simulink model "ISTrain_2024"  (R2024b)
settings: Solver=ode4  StartTime=0.0  StopTime=StopTime  FixedStep=StepSize  RelTol=1e-3
undefined symbols (not defined in the file or in its folder): Crr, eta_mech, g, G, grade, LM, LMatrix, LR, m_loco, m_total, maxID, maxIQ, maxTorque, Pp, r_w, RLInv, Rr
libraries: slpidlib x3
settings Model: Creator=rafae  LastModifiedBy=rafae

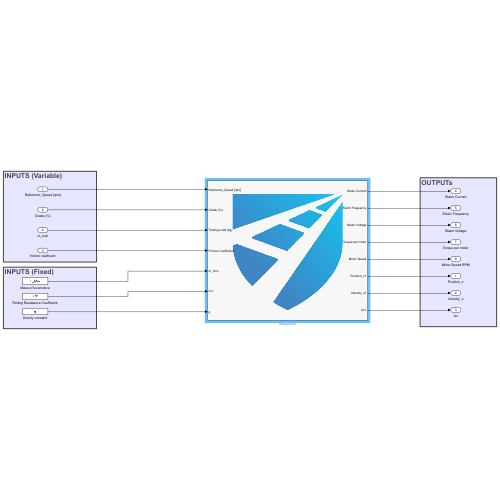
[thumbnail: Simulink's stored preview of the top-level diagram]
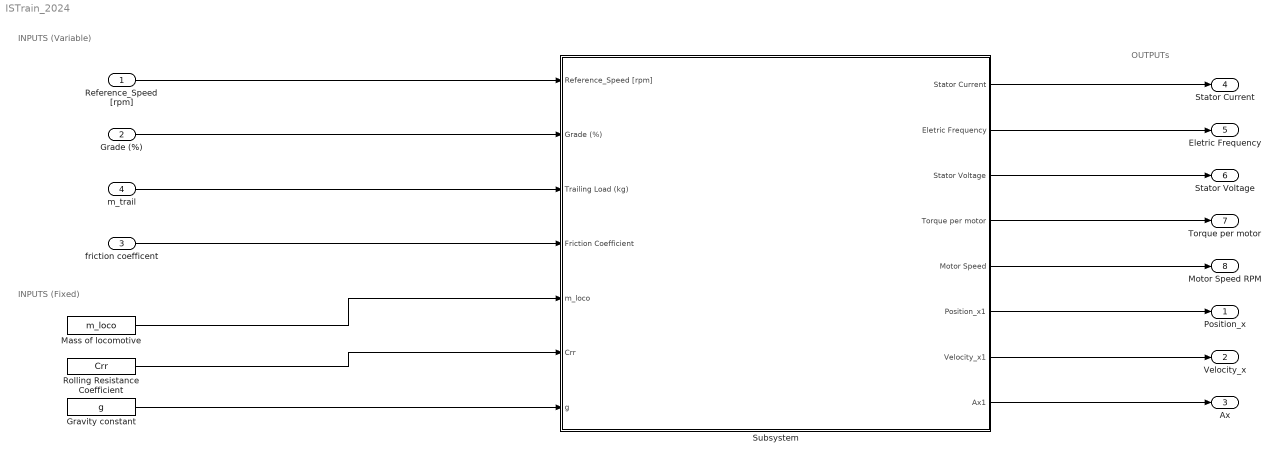
== system ISTrain_2024 ==
  note: OUTPUTs
  note: INPUTS (Variable)
  note: INPUTS (Fixed)
  Reference_Speed [rpm] : Inport
  Grade (%) : Inport  Port=2
  friction coefficent : Inport  Port=3
  m_trail : Inport  Port=4
  Gravity constant : Constant  Value=g
  Mass of locomotive : Constant  Value=m_loco
  Rolling Resistance Coefficient : Constant  Value=Crr
  Subsystem : Subsystem
      mask Display: image('ist_train_logo.jpg');
  Position_x : Outport
  Velocity_x : Outport  Port=2
  Ax : Outport  Port=3
  Stator Current : Outport  Port=4
  Eletric Frequency : Outport  Port=5
  Stator Voltage : Outport  Port=6
  Torque per motor : Outport  Port=7
  Motor Speed RPM : Outport  Port=8
  wires:
  Reference_Speed [rpm]/1 -> Subsystem/1(Reference_Speed [rpm])
  Subsystem/6(Position_x1) -> Position_x/1
  Subsystem/7(Velocity_x1) -> Velocity_x/1
  Subsystem/8(Ax1) -> Ax/1
  Subsystem/1(Stator Current) -> Stator Current/1
  Subsystem/2(Eletric Frequency) -> Eletric Frequency/1
  Subsystem/3(Stator Voltage) -> Stator Voltage/1
  Subsystem/4(Torque per motor) -> Torque per motor/1
  Subsystem/5(Motor Speed) -> Motor Speed RPM/1
  Grade (%)/1 -> Subsystem/2(Grade (%))
  m_trail/1 -> Subsystem/3(Trailing Load (kg))
  friction coefficent/1 -> Subsystem/4(Friction Coefficient)
  Mass of locomotive/1 -> Subsystem/5(m_loco)
  Rolling Resistance Coefficient/1 -> Subsystem/6(Crr)
  Gravity constant/1 -> Subsystem/7(g)

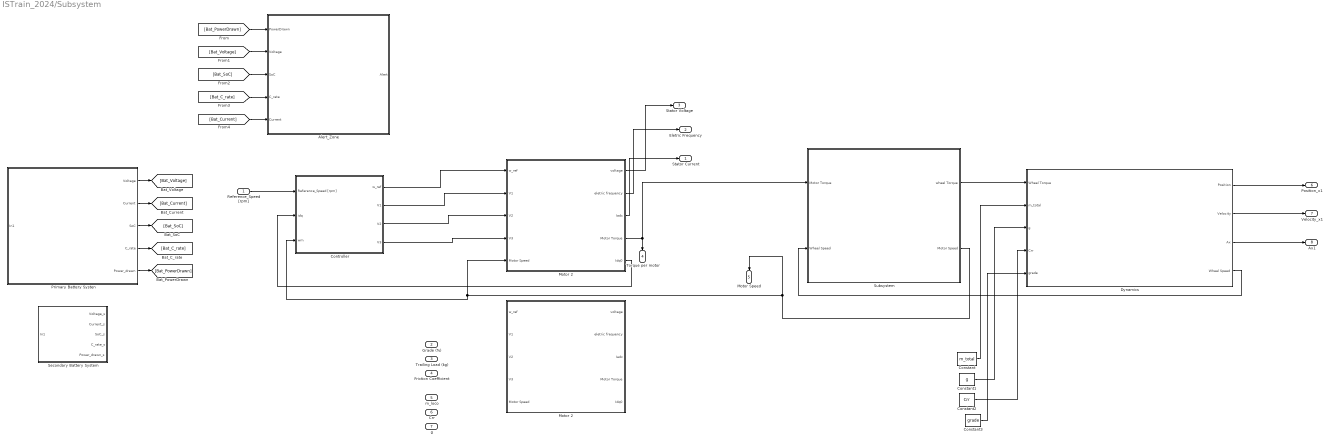
== system ISTrain_2024/Subsystem ==
  Reference_Speed [rpm] : Inport
  Grade (%) : Inport  Port=2
  Trailing Load (kg) : Inport  Port=3
  Friction Coefficient : Inport  Port=4
  m_loco : Inport  Port=5
  Crr : Inport  Port=6
  g : Inport  Port=7
  Alert_Zone : Subsystem
      mask Display: image('hazard.jpg');
  Constant : Constant  Value=m_total
  Constant1 : Constant  Value=g
  Constant2 : Constant  Value=Crr
  Constant3 : Constant  Value=grade
  Controller : Subsystem
      mask Display: image('motor controller.jpeg');
  Dynamics : Subsystem
      mask Display: image('wheel_train.jpg');
  Motor 2 : Subsystem
      mask Display: image('motor.jpg');
  "Motor 2 " : Subsystem
      mask Display: image('motor.jpg');
  Primary Battery Systen : Subsystem
      mask Display: image('battery system.png');
  Secondary Battery System : Subsystem
      mask Display: image('battery system.png');
  Subsystem : Subsystem
      mask Display: image('gear_system.png');
  Stator Current : Outport
  Eletric Frequency : Outport  Port=2
  Stator Voltage : Outport  Port=3
  Torque per motor : Outport  Port=4
  Motor Speed : Outport  Port=5
  Position_x1 : Outport  Port=6
  Velocity_x1 : Outport  Port=7
  Ax1 : Outport  Port=8
  wires:
  Reference_Speed [rpm]/1 -> Controller/1(Reference_Speed [rpm])
  Subsystem/2(Motor Speed) -> Motor Speed/1, Controller/3(wm), "Motor 2 "/5(Motor Speed)
  Dynamics/4(Wheel Speed) -> Subsystem/2(Wheel Speed)
  Controller/1(w_ref) -> "Motor 2 "/1(w_ref)
  Controller/2(V1) -> "Motor 2 "/2(V1)
  Controller/3(V2) -> "Motor 2 "/3(V2)
  Controller/4(V3) -> "Motor 2 "/4(V3)
  "Motor 2 "/5(Idq0) -> Controller/2(idq)
  "Motor 2 "/1(voltage) -> Stator Voltage/1
  "Motor 2 "/2(eletric frequency) -> Eletric Frequency/1
  "Motor 2 "/3(Iadc) -> Stator Current/1
  "Motor 2 "/4(Motor Torque) -> Subsystem/1(Motor Torque), Torque per motor/1
  Subsystem/1(wheel Torque) -> Dynamics/1(Wheel Torque)
  Constant3/1 -> Dynamics/5(grade)
  Constant1/1 -> Dynamics/3(g)
  Constant2/1 -> Dynamics/4(Crr)
  Constant/1 -> Dynamics/2(m_total)
  Dynamics/3(Ax) -> Ax1/1
  Dynamics/2(Velocity) -> Velocity_x1/1
  Dynamics/1(Position) -> Position_x1/1
  Primary Battery Systen/1(Voltage) -> [Bat_Voltage]
  Primary Battery Systen/2(Current) -> [Bat_Current]
  Primary Battery Systen/3(SoC) -> [Bat_SoC]
  Primary Battery Systen/5(Power_drawn) -> [Bat_PowerDrawn]
  Primary Battery Systen/4(C_rate) -> [Bat_C_rate]
  [Bat_Current] -> Alert_Zone/5(Current)
  [Bat_C_rate] -> Alert_Zone/4(C_rate)
  [Bat_SoC] -> Alert_Zone/3(SoC)
  [Bat_Voltage] -> Alert_Zone/2(Voltage)
  [Bat_PowerDrawn] -> Alert_Zone/1(PowerDrawn)

== system ISTrain_2024/Subsystem/Alert_Zone ==
  PowerDrawn : Inport
  Voltage : Inport  Port=2
  SoC : Inport  Port=3
  C_rate : Inport  Port=4
  Current : Inport  Port=5
  MATLAB Function : MATLAB Function  TreatAsAtomicUnit=on
  Alert : Outport
  wires:
  Voltage/1 -> MATLAB Function/2(Voltage)
  SoC/1 -> MATLAB Function/1(SoC)
  MATLAB Function/1(alert) -> Alert/1
  C_rate/1 -> MATLAB Function/3(C_rate)

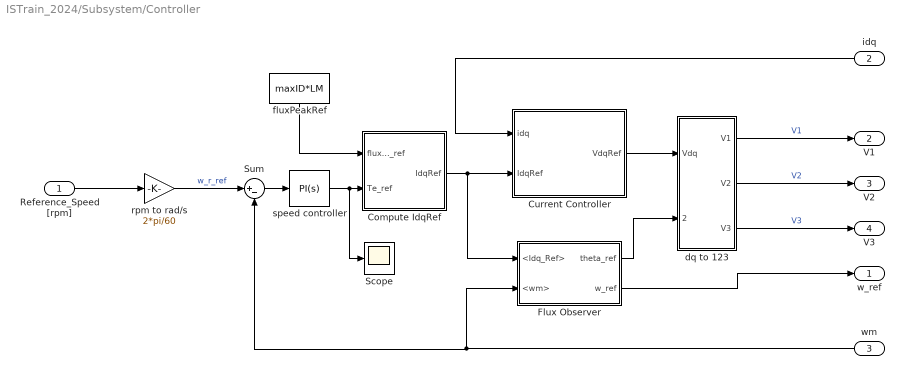
== system ISTrain_2024/Subsystem/Controller ==
  Reference_Speed [rpm] : Inport
  idq : Inport  Port=2
  wm : Inport  Port=3
  Compute IdqRef : Subsystem
  Current Controller : Subsystem
  Flux Observer : Subsystem
  Scope : Scope
  Sum : Sum  Inputs=|+-
  dq to 123 : Subsystem
  fluxPeakRef : Constant  Value=maxID*LM
  rpm to rad/s : Gain  Gain=2*pi/60
  speed controller : slpidlib/PID Controller  Controller=PI  Form=Parallel  TimeDomain=Continuous-time  UseExternalTs=off  SampleTime=-1  IntegratorMethod=Forward Euler  FilterMethod=Forward Euler  ControllerParametersSource=internal  P=50  I=100  UseKiTs=off  D=0  UseExternalDerivativeSource=off  N=100  UseFilter=on  TunerSelectOption=Transfer Function Based (PID Tuner App)  InitialConditionSource=internal  InitialConditionForIntegrator=0  InitialConditionForFilter=0  DifferentiatorICPrevScaledInput=0  ExternalReset=none  TrackingMode=off  Kt=1  LimitOutput=on  SatLimitsSource=internal  UpperSaturationLimit=maxTorque  LowerSaturationLimit=-maxTorque  LinearizeAsGain=on  AntiWindupMode=back-calculation  Kb=500  LimitIntegrator=off  UpperIntegratorSaturationLimit=inf  LowerIntegratorSaturationLimit=-inf  POutMin=[]  POutMax=[]  IOutMin=[]  IOutMax=[]  DOutMin=[]  DOutMax=[]  NOutMin=[]  NOutMax=[]  SumOutMin=[]  SumOutMax=[]  SaturationOutMin=[]  SaturationOutMax=[]  PParamMin=[]  PParamMax=[]  IParamMin=[]  IParamMax=[]  DParamMin=[]  DParamMax=[]  NParamMin=[]  NParamMax=[]  KbParamMin=[]  KbParamMax=[]  KtParamMin=[]  KtParamMax=[]  KbOutMin=[]  KbOutMax=[]  KtOutMin=[]  KtOutMax=[]  IntegratorOutMin=[]  IntegratorOutMax=[]  FilterOutMin=[]  FilterOutMax=[]  SumI1OutMin=[]  SumI1OutMax=[]  SumI2OutMin=[]  SumI2OutMax=[]  SumI3OutMin=[]  SumI3OutMax=[]  SumI4OutMin=[]  SumI4OutMax=[]  SumDOutMin=[]  SumDOutMax=[]  DifferentiatorOutMin=[]  DifferentiatorOutMax=[]  FilterDiffOutCoefMin=[]  FilterDiffOutCoefMax=[]  ReciprocalOutMin=[]  ReciprocalOutMax=[]  SumDenOutMin=[]  SumDenOutMax=[]  SumNumOutMin=[]  SumNumOutMax=[]  DivideOutMin=[]  DivideOutMax=[]  UdiffTsProdOutMin=[]  UdiffTsProdOutMax=[]  NTsProdOutMin=[]  NTsProdOutMax=[]  UintegralTsProdOutMin=[]  UintegralTsProdOutMax=[]  UngainTsProdOutMin=[]  UngainTsProdOutMax=[]  ClampingZeroOutDataTypeStr=Inherit: Inherit via back propagation  ClampingZeroOutMin=[]  ClampingZeroOutMax=[]  FilterDenConstantOutDataTypeStr=Inherit: Inherit via back propagation  FilterDenConstantOutMin=[]  FilterDenConstantOutMax=[]  PCopyOutDataTypeStr=Inherit: Inherit via back propagation  PCopyOutMin=[]  PCopyOutMax=[]  NCopyOutDataTypeStr=Inherit: Inherit via back propagation  NCopyOutMin=[]  NCopyOutMax=[]  IntegratorContinuousStateAttributes=''  IntegratorStateMustResolveToSignalObject=off  IntegratorRTWStateStorageClass=Auto  FilterContinuousStateAttributes=''  FilterStateMustResolveToSignalObject=off  FilterRTWStateStorageClass=Auto  ParallelPVariant=InternalParameters  IdealPVariant=Disabled  IVariant=InternalParameters  DVariant=Disabled  IntegratorVariant=Continuous  SatVariant=Enabled  AWVariant=BackCalculation  PCopyVariant=Disabled  TRVariant=Disabled  FdbkBlocksVariant=Forward  IdealPFdbkVariant=Disabled  SatFdbkVariant=Disabled  DerivativeFilterVariant=Disabled  NVariant=Disabled  NCopyVariant=Disabled_SignalSpec  FilterICVariant=Disabled  IntegratorICVariant=InternalICs  ExternalResetVariant=Disabled  TRSumVariant=Passthrough  SumFdbkVariant=Disabled  SumVariant=Sum_PI  TsampFilterVariant=InternalTs  TsampNgainVariant=Passthrough  TsampIntegralVariant=Disabled_SignalSpec  ExternalSaturationOutDataTypeStr=Inherit: Same as second input  DerivativeSourceVariant=Disabled  PreIntVariant=InternalPreInt
  w_ref : Outport  VectorParamsAs1DForOutWhenUnconnected=off
  V1 : Outport  Port=2  VectorParamsAs1DForOutWhenUnconnected=off
  V2 : Outport  Port=3  VectorParamsAs1DForOutWhenUnconnected=off
  V3 : Outport  Port=4  VectorParamsAs1DForOutWhenUnconnected=off
  wires:
  Compute IdqRef/1(IdqRef) -> Flux Observer/1(<Idq_Ref>), Current Controller/2(IdqRef)
  Sum/1 -> speed controller/1
  fluxPeakRef/1 -> Compute IdqRef/1(fluxdR_ref)
  dq to 123/3(V3) -> V3/1  "V3"
  wm/1 -> Sum/2, Flux Observer/2(<wm>)
  speed controller/1 -> Scope/1, Compute IdqRef/2(Te_ref)
  idq/1 -> Current Controller/1(idq)
  Reference_Speed [rpm]/1 -> rpm to rad/s/1
  dq to 123/2(V2) -> V2/1  "V2"
  dq to 123/1(V1) -> V1/1  "V1"
  rpm to rad/s/1 -> Sum/1  "w_r_ref"
  Flux Observer/2(w_ref) -> w_ref/1
  Flux Observer/1(theta_ref) -> dq to 123/2(theta_ref)
  Current Controller/1(VdqRef) -> dq to 123/1(Vdq)

== system ISTrain_2024/Subsystem/Dynamics ==
  Wheel Torque : Inport
  m_total : Inport  Port=2
  g : Inport  Port=3
  Crr : Inport  Port=4
  grade : Inport  Port=5
  Gain : Gain  Gain=1/(m_total)
  Gain1 : Gain  Gain=1/r_w
  Integrator : Integrator
  Integrator1 : Integrator
  MATLAB Function : MATLAB Function  TreatAsAtomicUnit=on
  Subtract : Sum  Inputs=+-
  Position : Outport
  Velocity : Outport  Port=2
  Ax : Outport  Port=3
  Wheel Speed : Outport  Port=4
  wires:
  Integrator1/1 -> Position/1
  grade/1 -> MATLAB Function/4(grade)
  Crr/1 -> MATLAB Function/3(Crr)
  Subtract/1 -> Gain/1
  Integrator/1 -> Gain1/1, Velocity/1, Integrator1/1
  MATLAB Function/1(F_res) -> Subtract/2
  m_total/1 -> MATLAB Function/1(m_total)
  g/1 -> MATLAB Function/2(g)
  Gain1/1 -> Wheel Speed/1
  Gain/1 -> Ax/1, Integrator/1
  Wheel Torque/1 -> Subtract/1

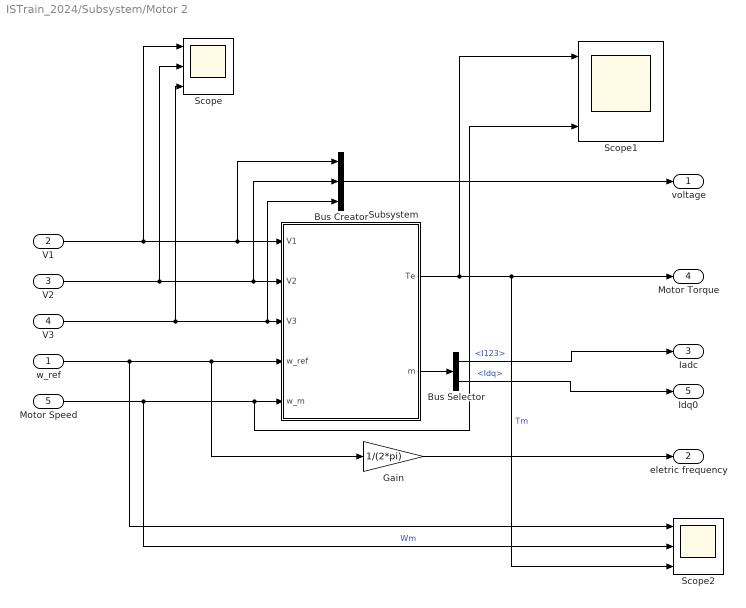
== system ISTrain_2024/Subsystem/Motor 2 ==
  w_ref : Inport
  V1 : Inport  Port=2
  V2 : Inport  Port=3
  V3 : Inport  Port=4
  Motor Speed : Inport  Port=5
  Bus Creator : BusCreator  Inputs=3
  Bus Selector : BusSelector  OutputSignals=I123,Idq
  Gain : Gain  Gain=1/(2*pi)
  Scope : Scope  NumInputPorts=3
  Scope1 : Scope  NumInputPorts=3
  Scope2 : Scope  NumInputPorts=3
  Subsystem : Subsystem
  voltage : Outport  VectorParamsAs1DForOutWhenUnconnected=off
  eletric frequency : Outport  Port=2  VectorParamsAs1DForOutWhenUnconnected=off
  Iadc : Outport  Port=3  VectorParamsAs1DForOutWhenUnconnected=off
  Motor Torque : Outport  Port=4  VectorParamsAs1DForOutWhenUnconnected=off
  Idq0 : Outport  Port=5  VectorParamsAs1DForOutWhenUnconnected=off
  wires:
  Gain/1 -> eletric frequency/1
  Subsystem/1(Te) -> Scope1/1, Scope2/3, Motor Torque/1  "Tm"
  Bus Selector/2 -> Idq0/1  "<Idq>"
  Subsystem/2(m) -> Bus Selector/1
  Bus Creator/1 -> voltage/1
  V1/1 -> Bus Creator/1, Subsystem/1(V1), Scope/1
  Motor Speed/1 -> Scope2/2, Scope1/3, Subsystem/5(w_m)  "Wm"
  Bus Selector/1 -> Iadc/1  "<I123>"
  w_ref/1 -> Scope2/1, Gain/1, Subsystem/4(w_ref)
  V2/1 -> Bus Creator/2, Subsystem/2(V2), Scope/2
  V3/1 -> Scope/3, Bus Creator/3, Subsystem/3(V3)

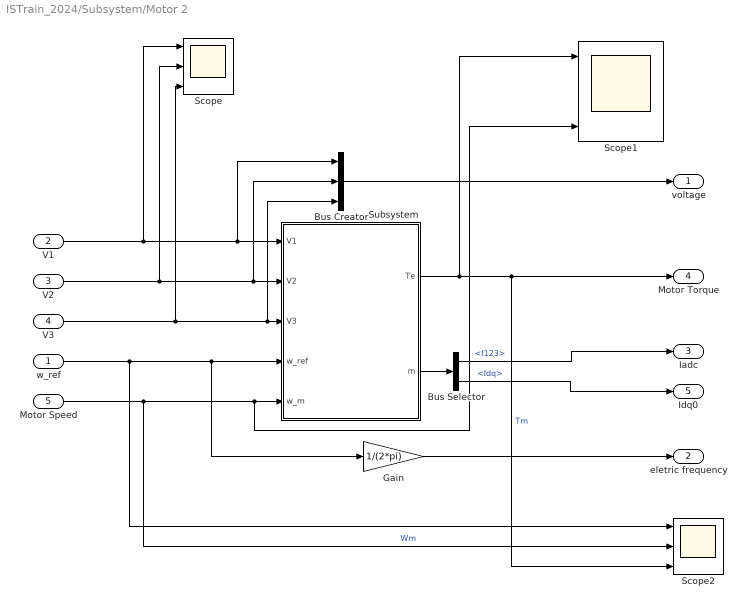
== system ISTrain_2024/Subsystem/Motor 2  ==
  w_ref : Inport
  V1 : Inport  Port=2
  V2 : Inport  Port=3
  V3 : Inport  Port=4
  Motor Speed : Inport  Port=5
  Bus Creator : BusCreator  Inputs=3
  Bus Selector : BusSelector  OutputSignals=I123,Idq
  Gain : Gain  Gain=1/(2*pi)
  Scope : Scope  NumInputPorts=3
  Scope1 : Scope  NumInputPorts=3
  Scope2 : Scope  NumInputPorts=3
  Subsystem : Subsystem
  voltage : Outport  VectorParamsAs1DForOutWhenUnconnected=off
  eletric frequency : Outport  Port=2  VectorParamsAs1DForOutWhenUnconnected=off
  Iadc : Outport  Port=3  VectorParamsAs1DForOutWhenUnconnected=off
  Motor Torque : Outport  Port=4  VectorParamsAs1DForOutWhenUnconnected=off
  Idq0 : Outport  Port=5  VectorParamsAs1DForOutWhenUnconnected=off
  wires:
  Gain/1 -> eletric frequency/1
  Subsystem/1(Te) -> Scope1/1, Scope2/3, Motor Torque/1  "Tm"
  Bus Selector/2 -> Idq0/1  "<Idq>"
  Subsystem/2(m) -> Bus Selector/1
  Bus Creator/1 -> voltage/1
  V1/1 -> Bus Creator/1, Subsystem/1(V1), Scope/1
  Motor Speed/1 -> Scope2/2, Scope1/3, Subsystem/5(w_m)  "Wm"
  Bus Selector/1 -> Iadc/1  "<I123>"
  w_ref/1 -> Scope2/1, Gain/1, Subsystem/4(w_ref)
  V2/1 -> Bus Creator/2, Subsystem/2(V2), Scope/2
  V3/1 -> Scope/3, Bus Creator/3, Subsystem/3(V3)

== system ISTrain_2024/Subsystem/Primary Battery Systen ==
  In1 : Inport
  From Workspace : FromWorkspace  VariableName=power_signal
  MATLAB Function : MATLAB Function  TreatAsAtomicUnit=on
  Scope : Scope  NumInputPorts=5
  Voltage : Outport
  Current : Outport  Port=2
  SoC : Outport  Port=3
  C_rate : Outport  Port=4
  Power_drawn : Outport  Port=5
  wires:
  From Workspace/1 -> MATLAB Function/1(P_in)
  MATLAB Function/1(V_out) -> Scope/1, Voltage/1
  MATLAB Function/2(I_out) -> Scope/2, Current/1
  MATLAB Function/3(SoC_out) -> Scope/3, SoC/1
  MATLAB Function/4(C_out) -> Scope/4, C_rate/1
  MATLAB Function/5(P_out) -> Scope/5, Power_drawn/1

== system ISTrain_2024/Subsystem/Secondary Battery System ==
  In1 : Inport
  Voltage_s : Outport
  Current_s : Outport  Port=2
  SoC_s : Outport  Port=3
  C_rate_s : Outport  Port=4
  Power_drawn_s : Outport  Port=5

== system ISTrain_2024/Subsystem/Subsystem ==
  Motor Torque : Inport
  Wheel Speed : Inport  Port=2
  GearBox : Subsystem
  wheel Torque : Outport
  Motor Speed : Outport  Port=2
  wires:
  Motor Torque/1 -> GearBox/1(Torque total)
  Wheel Speed/1 -> Motor Speed/1
  GearBox/1(Tractive_Force) -> wheel Torque/1

== system ISTrain_2024/Subsystem/Controller/Compute IdqRef ==
  fluxdR_ref : Inport
  Te_ref : Inport  Port=2
  Fcn : Fcn  Expr=u(2)/(3/2*Pp*(LM/LR)*u(1))
  Gain : Gain  Gain=1/LM
  Mux : Mux  Inputs=2
  Mux1 : Mux  Inputs=2
  Saturation : Saturate  UpperLimit=maxID  LowerLimit=-maxID
  Saturation1 : Saturate  UpperLimit=maxIQ  LowerLimit=-maxIQ
  IdqRef : Outport  VectorParamsAs1DForOutWhenUnconnected=off
  wires:
  fluxdR_ref/1 -> Mux/1, Gain/1
  Mux/1 -> Fcn/1
  Fcn/1 -> Saturation1/1
  Gain/1 -> Saturation/1
  Mux1/1 -> IdqRef/1
  Te_ref/1 -> Mux/2
  Saturation/1 -> Mux1/1  "id"
  Saturation1/1 -> Mux1/2  "iq"

== system ISTrain_2024/Subsystem/Controller/Current Controller ==
  idq : Inport
  IdqRef : Inport  Port=2
  Demux : Demux  Outputs=2
  Mux : Mux  Inputs=2
  PID Controller : slpidlib/PID Controller  Controller=PI  Form=Parallel  TimeDomain=Continuous-time  UseExternalTs=off  SampleTime=-1  IntegratorMethod=Forward Euler  FilterMethod=Forward Euler  ControllerParametersSource=internal  P=5  I=100  UseKiTs=off  D=0  UseExternalDerivativeSource=off  N=100  UseFilter=on  TunerSelectOption=Transfer Function Based (PID Tuner App)  InitialConditionSource=internal  InitialConditionForIntegrator=0  InitialConditionForFilter=0  DifferentiatorICPrevScaledInput=0  ExternalReset=none  TrackingMode=off  Kt=1  LimitOutput=on  SatLimitsSource=internal  UpperSaturationLimit=600  LowerSaturationLimit=-600  LinearizeAsGain=on  AntiWindupMode=back-calculation  Kb=1  LimitIntegrator=off  UpperIntegratorSaturationLimit=inf  LowerIntegratorSaturationLimit=-inf  POutMin=[]  POutMax=[]  IOutMin=[]  IOutMax=[]  DOutMin=[]  DOutMax=[]  NOutMin=[]  NOutMax=[]  SumOutMin=[]  SumOutMax=[]  SaturationOutMin=[]  SaturationOutMax=[]  PParamMin=[]  PParamMax=[]  IParamMin=[]  IParamMax=[]  DParamMin=[]  DParamMax=[]  NParamMin=[]  NParamMax=[]  KbParamMin=[]  KbParamMax=[]  KtParamMin=[]  KtParamMax=[]  KbOutMin=[]  KbOutMax=[]  KtOutMin=[]  KtOutMax=[]  IntegratorOutMin=[]  IntegratorOutMax=[]  FilterOutMin=[]  FilterOutMax=[]  SumI1OutMin=[]  SumI1OutMax=[]  SumI2OutMin=[]  SumI2OutMax=[]  SumI3OutMin=[]  SumI3OutMax=[]  SumI4OutMin=[]  SumI4OutMax=[]  SumDOutMin=[]  SumDOutMax=[]  DifferentiatorOutMin=[]  DifferentiatorOutMax=[]  FilterDiffOutCoefMin=[]  FilterDiffOutCoefMax=[]  ReciprocalOutMin=[]  ReciprocalOutMax=[]  SumDenOutMin=[]  SumDenOutMax=[]  SumNumOutMin=[]  SumNumOutMax=[]  DivideOutMin=[]  DivideOutMax=[]  UdiffTsProdOutMin=[]  UdiffTsProdOutMax=[]  NTsProdOutMin=[]  NTsProdOutMax=[]  UintegralTsProdOutMin=[]  UintegralTsProdOutMax=[]  UngainTsProdOutMin=[]  UngainTsProdOutMax=[]  ClampingZeroOutDataTypeStr=Inherit: Inherit via back propagation  ClampingZeroOutMin=[]  ClampingZeroOutMax=[]  FilterDenConstantOutDataTypeStr=Inherit: Inherit via back propagation  FilterDenConstantOutMin=[]  FilterDenConstantOutMax=[]  PCopyOutDataTypeStr=Inherit: Inherit via back propagation  PCopyOutMin=[]  PCopyOutMax=[]  NCopyOutDataTypeStr=Inherit: Inherit via back propagation  NCopyOutMin=[]  NCopyOutMax=[]  IntegratorContinuousStateAttributes=''  IntegratorStateMustResolveToSignalObject=off  IntegratorRTWStateStorageClass=Auto  FilterContinuousStateAttributes=''  FilterStateMustResolveToSignalObject=off  FilterRTWStateStorageClass=Auto  ParallelPVariant=InternalParameters  IdealPVariant=Disabled  IVariant=InternalParameters  DVariant=Disabled  IntegratorVariant=Continuous  SatVariant=Enabled  AWVariant=BackCalculation  PCopyVariant=Disabled  TRVariant=Disabled  FdbkBlocksVariant=Forward  IdealPFdbkVariant=Disabled  SatFdbkVariant=Disabled  DerivativeFilterVariant=Disabled  NVariant=Disabled  NCopyVariant=Disabled_SignalSpec  FilterICVariant=Disabled  IntegratorICVariant=InternalICs  ExternalResetVariant=Disabled  TRSumVariant=Passthrough  SumFdbkVariant=Disabled  SumVariant=Sum_PI  TsampFilterVariant=InternalTs  TsampNgainVariant=Passthrough  TsampIntegralVariant=Disabled_SignalSpec  ExternalSaturationOutDataTypeStr=Inherit: Same as second input  DerivativeSourceVariant=Disabled  PreIntVariant=InternalPreInt
  PID Controller1 : slpidlib/PID Controller  Controller=PI  Form=Parallel  TimeDomain=Continuous-time  UseExternalTs=off  SampleTime=-1  IntegratorMethod=Forward Euler  FilterMethod=Forward Euler  ControllerParametersSource=internal  P=5  I=100  UseKiTs=off  D=0  UseExternalDerivativeSource=off  N=100  UseFilter=on  TunerSelectOption=Transfer Function Based (PID Tuner App)  InitialConditionSource=internal  InitialConditionForIntegrator=0  InitialConditionForFilter=0  DifferentiatorICPrevScaledInput=0  ExternalReset=none  TrackingMode=off  Kt=1  LimitOutput=on  SatLimitsSource=internal  UpperSaturationLimit=600  LowerSaturationLimit=-600  LinearizeAsGain=on  AntiWindupMode=back-calculation  Kb=1  LimitIntegrator=off  UpperIntegratorSaturationLimit=inf  LowerIntegratorSaturationLimit=-inf  POutMin=[]  POutMax=[]  IOutMin=[]  IOutMax=[]  DOutMin=[]  DOutMax=[]  NOutMin=[]  NOutMax=[]  SumOutMin=[]  SumOutMax=[]  SaturationOutMin=[]  SaturationOutMax=[]  PParamMin=[]  PParamMax=[]  IParamMin=[]  IParamMax=[]  DParamMin=[]  DParamMax=[]  NParamMin=[]  NParamMax=[]  KbParamMin=[]  KbParamMax=[]  KtParamMin=[]  KtParamMax=[]  KbOutMin=[]  KbOutMax=[]  KtOutMin=[]  KtOutMax=[]  IntegratorOutMin=[]  IntegratorOutMax=[]  FilterOutMin=[]  FilterOutMax=[]  SumI1OutMin=[]  SumI1OutMax=[]  SumI2OutMin=[]  SumI2OutMax=[]  SumI3OutMin=[]  SumI3OutMax=[]  SumI4OutMin=[]  SumI4OutMax=[]  SumDOutMin=[]  SumDOutMax=[]  DifferentiatorOutMin=[]  DifferentiatorOutMax=[]  FilterDiffOutCoefMin=[]  FilterDiffOutCoefMax=[]  ReciprocalOutMin=[]  ReciprocalOutMax=[]  SumDenOutMin=[]  SumDenOutMax=[]  SumNumOutMin=[]  SumNumOutMax=[]  DivideOutMin=[]  DivideOutMax=[]  UdiffTsProdOutMin=[]  UdiffTsProdOutMax=[]  NTsProdOutMin=[]  NTsProdOutMax=[]  UintegralTsProdOutMin=[]  UintegralTsProdOutMax=[]  UngainTsProdOutMin=[]  UngainTsProdOutMax=[]  ClampingZeroOutDataTypeStr=Inherit: Inherit via back propagation  ClampingZeroOutMin=[]  ClampingZeroOutMax=[]  FilterDenConstantOutDataTypeStr=Inherit: Inherit via back propagation  FilterDenConstantOutMin=[]  FilterDenConstantOutMax=[]  PCopyOutDataTypeStr=Inherit: Inherit via back propagation  PCopyOutMin=[]  PCopyOutMax=[]  NCopyOutDataTypeStr=Inherit: Inherit via back propagation  NCopyOutMin=[]  NCopyOutMax=[]  IntegratorContinuousStateAttributes=''  IntegratorStateMustResolveToSignalObject=off  IntegratorRTWStateStorageClass=Auto  FilterContinuousStateAttributes=''  FilterStateMustResolveToSignalObject=off  FilterRTWStateStorageClass=Auto  ParallelPVariant=InternalParameters  IdealPVariant=Disabled  IVariant=InternalParameters  DVariant=Disabled  IntegratorVariant=Continuous  SatVariant=Enabled  AWVariant=BackCalculation  PCopyVariant=Disabled  TRVariant=Disabled  FdbkBlocksVariant=Forward  IdealPFdbkVariant=Disabled  SatFdbkVariant=Disabled  DerivativeFilterVariant=Disabled  NVariant=Disabled  NCopyVariant=Disabled_SignalSpec  FilterICVariant=Disabled  IntegratorICVariant=InternalICs  ExternalResetVariant=Disabled  TRSumVariant=Passthrough  SumFdbkVariant=Disabled  SumVariant=Sum_PI  TsampFilterVariant=InternalTs  TsampNgainVariant=Passthrough  TsampIntegralVariant=Disabled_SignalSpec  ExternalSaturationOutDataTypeStr=Inherit: Same as second input  DerivativeSourceVariant=Disabled  PreIntVariant=InternalPreInt
  Scope2 : Scope  NumInputPorts=2
  Sum1 : Sum  Inputs=+-
  VdqRef : Outport  VectorParamsAs1DForOutWhenUnconnected=off
  wires:
  IdqRef/1 -> Scope2/1, Sum1/1
  idq/1 -> Sum1/2
  PID Controller/1 -> Mux/1  "PI"
  Sum1/1 -> Scope2/2, Demux/1  "error"
  Demux/1 -> PID Controller/1
  Demux/2 -> PID Controller1/1
  PID Controller1/1 -> Mux/2
  Mux/1 -> VdqRef/1

== system ISTrain_2024/Subsystem/Controller/Flux Observer ==
  <Idq_Ref> : Inport
  <wm> : Inport  Port=2
  Add : Sum  Inputs=2
  Bias : Bias  Bias=+eps  SaturateOnIntegerOverflow=off
  Constant1 : Constant  Value=1/(LR/Rr)
  Demux : Demux  Outputs=2
  Gain : Gain  Gain=Pp
  Integrator : Integrator
  Product : Product  Inputs=*/
  Product1 : Product
  Selector : Selector  InputPortWidth=2  IndexOptions=Index vector (dialog)  Indices=[2 1]  OutputSizes=1
  theta_ref : Outport  VectorParamsAs1DForOutWhenUnconnected=off
  w_ref : Outport  Port=2  VectorParamsAs1DForOutWhenUnconnected=off
  wires:
  Demux/1 -> Product/1
  <wm>/1 -> Gain/1
  Constant1/1 -> Product1/1
  Selector/1 -> Demux/1
  Product1/1 -> Add/2
  Product/1 -> Product1/2
  <Idq_Ref>/1 -> Selector/1
  Add/1 -> w_ref/1, Integrator/1
  Bias/1 -> Product/2
  Demux/2 -> Bias/1
  Integrator/1 -> theta_ref/1
  Gain/1 -> Add/1

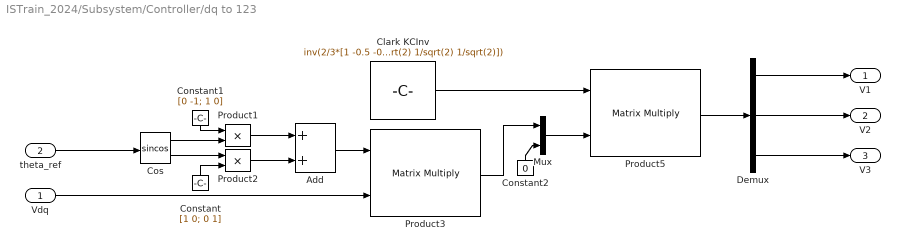
== system ISTrain_2024/Subsystem/Controller/dq to 123 ==
  Vdq : Inport
  theta_ref : Inport  Port=2
  Add : Sum
  Clark KCInv : Constant  Value=inv(2/3*[1 -0.5 -0.5; 0 sqrt(3)/2 -sqrt(3)/2; 1/sqrt(2) 1/sqrt(2) 1/sqrt(2)])
  Constant : Constant  Value=[1 0; 0 1]
  Constant1 : Constant  Value=[0 -1; 1 0]
  Constant2 : Constant  Value=0
  Cos : Trigonometry  Operator=sincos
  Demux : Demux  Outputs=3
  Mux : Mux  Inputs=2
  Product1 : Product
  Product2 : Product
  Product3 : Product  Multiplication=Matrix(*)
  Product5 : Product  Multiplication=Matrix(*)
  V1 : Outport  VectorParamsAs1DForOutWhenUnconnected=off
  V2 : Outport  Port=2  VectorParamsAs1DForOutWhenUnconnected=off
  V3 : Outport  Port=3  VectorParamsAs1DForOutWhenUnconnected=off
  wires:
  Cos/1 -> Product1/2
  Constant1/1 -> Product1/1
  Product2/1 -> Add/2
  Cos/2 -> Product2/1
  Product1/1 -> Add/1
  Constant/1 -> Product2/2
  Add/1 -> Product3/1
  Product3/1 -> Mux/1
  Clark KCInv/1 -> Product5/1
  Mux/1 -> Product5/2
  Constant2/1 -> Mux/2
  Vdq/1 -> Product3/2
  Demux/1 -> V1/1
  Demux/2 -> V2/1
  Demux/3 -> V3/1
  Product5/1 -> Demux/1
  theta_ref/1 -> Cos/1

== system ISTrain_2024/Subsystem/Motor 2/Subsystem ==
  note: V1 - phase-to-neutral voltage of phase 1 [V]
      | V2 - phase-to-neutral voltage of phase 2 [V]
      | V3 - phase-to-neutral voltage of phase 3 [V]
      | w_ref - reference of dq transformation (synchornous electric speed in this case = 2*pi*f) [rad/s]
      | w_m - motor angular speed [rad/s]
  V1 : Inport
  V2 : Inport  Port=2
  V3 : Inport  Port=3
  w_ref : Inport  Port=4
  w_m : Inport  Port=5
  Induction Machine Model : Subsystem
  Te : Outport  VectorParamsAs1DForOutWhenUnconnected=off
  m : Outport  Port=2  VectorParamsAs1DForOutWhenUnconnected=off
  wires:
  Induction Machine Model/1(m) -> m/1
  w_ref/1 -> Induction Machine Model/5(w_ref)
  V1/1 -> Induction Machine Model/2(V1)
  Induction Machine Model/2(Te) -> Te/1
  V2/1 -> Induction Machine Model/3(V2)
  V3/1 -> Induction Machine Model/4(V3)
  w_m/1 -> Induction Machine Model/1(wm)

== system ISTrain_2024/Subsystem/Motor 2 /Subsystem ==
  note: V1 - phase-to-neutral voltage of phase 1 [V]
      | V2 - phase-to-neutral voltage of phase 2 [V]
      | V3 - phase-to-neutral voltage of phase 3 [V]
      | w_ref - reference of dq transformation (synchornous electric speed in this case = 2*pi*f) [rad/s]
      | w_m - motor angular speed [rad/s]
  V1 : Inport
  V2 : Inport  Port=2
  V3 : Inport  Port=3
  w_ref : Inport  Port=4
  w_m : Inport  Port=5
  Induction Machine Model : Subsystem
  Te : Outport  VectorParamsAs1DForOutWhenUnconnected=off
  m : Outport  Port=2  VectorParamsAs1DForOutWhenUnconnected=off
  wires:
  Induction Machine Model/1(m) -> m/1
  w_ref/1 -> Induction Machine Model/5(w_ref)
  V1/1 -> Induction Machine Model/2(V1)
  Induction Machine Model/2(Te) -> Te/1
  V2/1 -> Induction Machine Model/3(V2)
  V3/1 -> Induction Machine Model/4(V3)
  w_m/1 -> Induction Machine Model/1(wm)

== system ISTrain_2024/Subsystem/Subsystem/GearBox ==
  Torque total : Inport
  Gear_ratio : Gain  Gain=G
  eta_mech : Gain  Gain=eta_mech
  Tractive_Force : Outport
  wires:
  Gear_ratio/1 -> eta_mech/1
  Torque total/1 -> Gear_ratio/1
  eta_mech/1 -> Tractive_Force/1

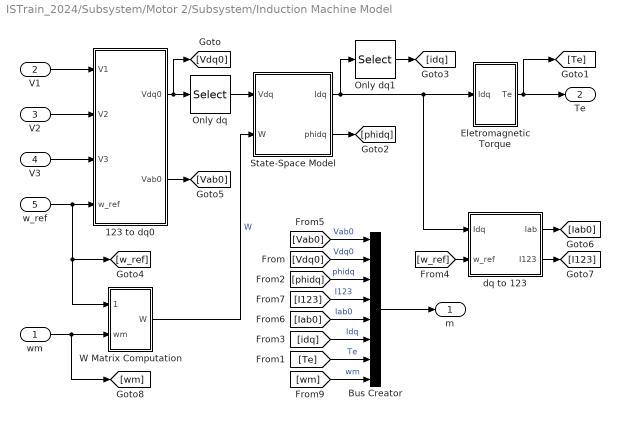
== system ISTrain_2024/Subsystem/Motor 2/Subsystem/Induction Machine Model ==
  wm : Inport
  V1 : Inport  Port=2
  V2 : Inport  Port=3
  V3 : Inport  Port=4
  w_ref : Inport  Port=5
  123 to dq0 : Subsystem
  Bus Creator : BusCreator  Inputs=8
  Eletromagnetic Torque : Subsystem
  Only dq : Selector  InputPortWidth=3  IndexOptions=Index vector (dialog)  Indices=[1 2]  OutputSizes=1
  Only dq1 : Selector  InputPortWidth=4  IndexOptions=Index vector (dialog)  Indices=[1 2]  OutputSizes=1
  State-Space Model : Subsystem
  W Matrix Computation : Subsystem
  dq to 123 : Subsystem
  m : Outport  VectorParamsAs1DForOutWhenUnconnected=off
  Te : Outport  Port=2  VectorParamsAs1DForOutWhenUnconnected=off
  wires:
  123 to dq0/1(Vdq0) -> Only dq/1, [Vdq0]
  V3/1 -> 123 to dq0/3(V3)
  V2/1 -> 123 to dq0/2(V2)
  wm/1 -> [wm], W Matrix Computation/2(wm)
  123 to dq0/2(Vab0) -> [Vab0]
  W Matrix Computation/1(W) -> State-Space Model/2(W)  "W"
  Only dq/1 -> State-Space Model/1(Vdq)
  Eletromagnetic Torque/1(Te) -> Te/1, [Te]
  V1/1 -> 123 to dq0/1(V1)
  State-Space Model/1(Idq) -> dq to 123/1(Idq), Eletromagnetic Torque/1(Idq), Only dq1/1
  [w_ref] -> dq to 123/2(w_ref)
  State-Space Model/2(phidq) -> [phidq]
  dq to 123/1(Iab) -> [Iab0]
  dq to 123/2(I123) -> [I123]
  [Vab0] -> Bus Creator/1  "Vab0"
  [Vdq0] -> Bus Creator/2  "Vdq0"
  [phidq] -> Bus Creator/3  "phidq"
  [I123] -> Bus Creator/4  "I123"
  [Iab0] -> Bus Creator/5  "Iab0"
  [idq] -> Bus Creator/6  "Idq"
  [Te] -> Bus Creator/7  "Te"
  Bus Creator/1 -> m/1
  Only dq1/1 -> [idq]
  w_ref/1 -> 123 to dq0/4(w_ref), W Matrix Computation/1(w_ref), [w_ref]
  [wm] -> Bus Creator/8  "wm"

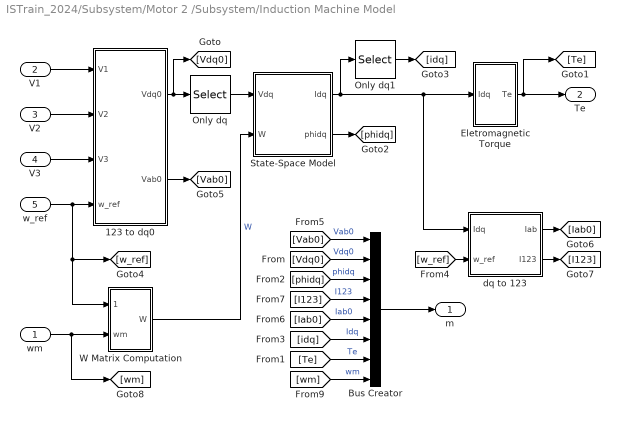
== system ISTrain_2024/Subsystem/Motor 2 /Subsystem/Induction Machine Model ==
  wm : Inport
  V1 : Inport  Port=2
  V2 : Inport  Port=3
  V3 : Inport  Port=4
  w_ref : Inport  Port=5
  123 to dq0 : Subsystem
  Bus Creator : BusCreator  Inputs=8
  Eletromagnetic Torque : Subsystem
  Only dq : Selector  InputPortWidth=3  IndexOptions=Index vector (dialog)  Indices=[1 2]  OutputSizes=1
  Only dq1 : Selector  InputPortWidth=4  IndexOptions=Index vector (dialog)  Indices=[1 2]  OutputSizes=1
  State-Space Model : Subsystem
  W Matrix Computation : Subsystem
  dq to 123 : Subsystem
  m : Outport  VectorParamsAs1DForOutWhenUnconnected=off
  Te : Outport  Port=2  VectorParamsAs1DForOutWhenUnconnected=off
  wires:
  123 to dq0/1(Vdq0) -> Only dq/1, [Vdq0]
  V3/1 -> 123 to dq0/3(V3)
  V2/1 -> 123 to dq0/2(V2)
  wm/1 -> [wm], W Matrix Computation/2(wm)
  123 to dq0/2(Vab0) -> [Vab0]
  W Matrix Computation/1(W) -> State-Space Model/2(W)  "W"
  Only dq/1 -> State-Space Model/1(Vdq)
  Eletromagnetic Torque/1(Te) -> Te/1, [Te]
  V1/1 -> 123 to dq0/1(V1)
  State-Space Model/1(Idq) -> dq to 123/1(Idq), Eletromagnetic Torque/1(Idq), Only dq1/1
  [w_ref] -> dq to 123/2(w_ref)
  State-Space Model/2(phidq) -> [phidq]
  dq to 123/1(Iab) -> [Iab0]
  dq to 123/2(I123) -> [I123]
  [Vab0] -> Bus Creator/1  "Vab0"
  [Vdq0] -> Bus Creator/2  "Vdq0"
  [phidq] -> Bus Creator/3  "phidq"
  [I123] -> Bus Creator/4  "I123"
  [Iab0] -> Bus Creator/5  "Iab0"
  [idq] -> Bus Creator/6  "Idq"
  [Te] -> Bus Creator/7  "Te"
  Bus Creator/1 -> m/1
  Only dq1/1 -> [idq]
  w_ref/1 -> 123 to dq0/4(w_ref), W Matrix Computation/1(w_ref), [w_ref]
  [wm] -> Bus Creator/8  "wm"

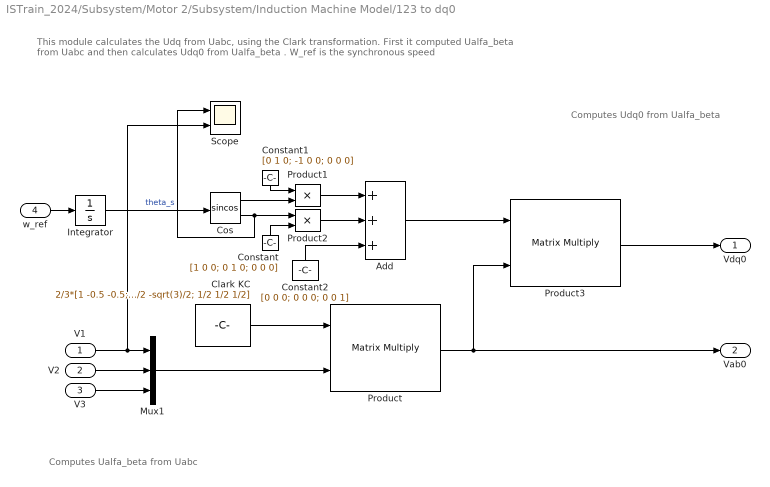
== system ISTrain_2024/Subsystem/Motor 2/Subsystem/Induction Machine Model/123 to dq0 ==
  note: Computes Ualfa_beta from Uabc
  note: This module calculates the Udq from Uabc, using the Clark transformation.
      | First it computed Ualfa_beta from Uabc and then calculates Udq0 from Ualfa_beta .
      | W_ref is the synchronous speed
  note: Computes Udq0 from Ualfa_beta
  V1 : Inport
  V2 : Inport  Port=2
  V3 : Inport  Port=3
  w_ref : Inport  Port=4
  Add : Sum  Inputs=+++
  Clark KC : Constant  Value=2/3*[1 -0.5 -0.5; 0 sqrt(3)/2 -sqrt(3)/2; 1/2 1/2 1/2]
  Constant : Constant  Value=[1 0 0; 0 1 0; 0 0 0]
  Constant1 : Constant  Value=[0 1 0; -1 0 0; 0 0 0]
  Constant2 : Constant  Value=[0 0 0; 0 0 0; 0 0 1]
  Cos : Trigonometry  Operator=sincos
  Integrator : Integrator
  Mux1 : Mux  Inputs=3
  Product : Product  Multiplication=Matrix(*)
  Product1 : Product
  Product2 : Product
  Product3 : Product  Multiplication=Matrix(*)
  Scope : Scope  NumInputPorts=2
  Vdq0 : Outport  VectorParamsAs1DForOutWhenUnconnected=off
  Vab0 : Outport  Port=2  VectorParamsAs1DForOutWhenUnconnected=off
  wires:
  Clark KC/1 -> Product/1
  Mux1/1 -> Product/2
  Product/1 -> Product3/2, Vab0/1
  Integrator/1 -> Cos/1  "theta_s"
  Cos/1 -> Product1/2
  Constant1/1 -> Product1/1
  Cos/2 -> Scope/1, Product2/1
  Constant/1 -> Product2/2
  Product1/1 -> Add/1
  Product2/1 -> Add/2
  Add/1 -> Product3/1
  Product3/1 -> Vdq0/1
  w_ref/1 -> Integrator/1
  Constant2/1 -> Add/3
  V2/1 -> Mux1/2
  V3/1 -> Mux1/3
  V1/1 -> Mux1/1, Scope/2

== system ISTrain_2024/Subsystem/Motor 2/Subsystem/Induction Machine Model/Eletromagnetic Torque ==
  Idq : Inport
  Constant : Constant  Value=3/2*LM*Pp
  Demux1 : Demux  Outputs=2
  Product : Product
  Product1 : Product  Inputs=1
  Product2 : Product  Inputs=1
  Selector : Selector  InputPortWidth=4  IndexOptions=Index vector (dialog)  Indices=[2 3 1 4]  OutputSizes=1
  Sum : Sum  Inputs=+-
  Te : Outport  VectorParamsAs1DForOutWhenUnconnected=off
  wires:
  Sum/1 -> Product/1
  Product1/1 -> Sum/1
  Demux1/1 -> Product1/1
  Product2/1 -> Sum/2
  Constant/1 -> Product/2
  Demux1/2 -> Product2/1
  Product/1 -> Te/1
  Idq/1 -> Selector/1
  Selector/1 -> Demux1/1

== system ISTrain_2024/Subsystem/Motor 2/Subsystem/Induction Machine Model/State-Space Model ==
  Vdq : Inport
  W : Inport  Port=2
  Constant : Constant  Value=RLInv  VectorParams1D=off
  Constant1 : Constant  Value=[0;0]
  Integrator : Integrator
  Linv : Constant  Value=inv(LMatrix)  VectorParams1D=off
  Product : Product  Multiplication=Matrix(*)
  Product1 : Product  Multiplication=Matrix(*)
  Sum : Sum  Inputs=|--
  Sum1 : Sum  Inputs=|++
  Vector Concatenate : Concatenate
  Idq : Outport  VectorParamsAs1DForOutWhenUnconnected=off
  phidq : Outport  Port=2  VectorParamsAs1DForOutWhenUnconnected=off
  wires:
  W/1 -> Sum/1
  Product/1 -> Sum1/2
  Constant/1 -> Sum/2
  Integrator/1 -> phidq/1, Product1/2, Product/2
  Product1/1 -> Idq/1
  Sum1/1 -> Integrator/1
  Sum/1 -> Product/1
  Linv/1 -> Product1/1
  Vdq/1 -> Vector Concatenate/1
  Constant1/1 -> Vector Concatenate/2
  Vector Concatenate/1 -> Sum1/1

== system ISTrain_2024/Subsystem/Motor 2/Subsystem/Induction Machine Model/W Matrix Computation ==
  note: computes W(dPsi/dt)=[0                     -d(theta_s)/dt          0                       0;
      |                                     d(theta_s)/dt           0                      0                      0;
      |                                    0                              0                      0             -d(theta_r)/dt;
      |                                    0                              0             d(theta_r)/dt              0;]
  w_ref : Inport
  wm : Inport  Port=2
  Gain : Gain  Gain=Pp
  Gain1 : Gain  Gain=-1  SaturateOnIntegerOverflow=on  OutDataTypeStr=Inherit: Same as input  ParamDataTypeStr=Inherit: Same as input
  Product : Product
  Sum2 : Sum  Inputs=-+|  InputSameDT=on  SaturateOnIntegerOverflow=on  OutDataTypeStr=Inherit: Same as first input
  W(3,4)=wr-1 : Assignment  NumberOfDimensions=2  IndexOptions=Index vector (dialog),Index vector (dialog)  Indices=3,4  OutputSizes=1,1
  W(4,3)=1-wr1 : Assignment  NumberOfDimensions=2  IndexOptions=Index vector (dialog),Index vector (dialog)  Indices=4,3  OutputSizes=1,1
  u1 : Constant  Value="[ 0 -1  0  0; 1  0  0  0;  0  0  0  0;  0  0  0  0]"
  W : Outport  InitialOutput=0  VectorParamsAs1DForOutWhenUnconnected=off
  wires:
  Gain1/1 -> W(3,4)=wr-1/2
  W(3,4)=wr-1/1 -> W/1
  Sum2/1 -> W(4,3)=1-wr1/2, Gain1/1  "we-w"
  wm/1 -> Gain/1
  W(4,3)=1-wr1/1 -> W(3,4)=wr-1/1
  Gain/1 -> Sum2/1
  w_ref/1 -> Product/1, Sum2/2
  u1/1 -> Product/2
  Product/1 -> W(4,3)=1-wr1/1

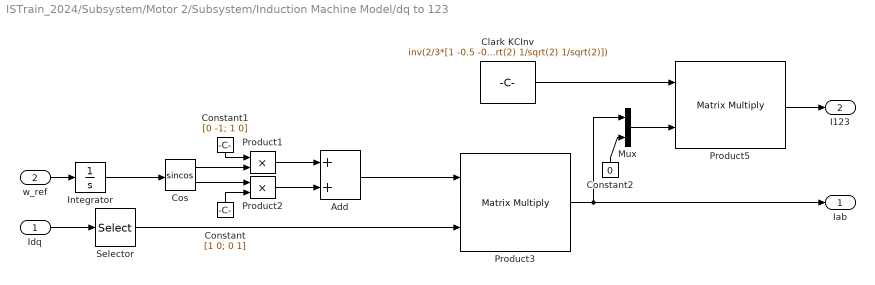
== system ISTrain_2024/Subsystem/Motor 2/Subsystem/Induction Machine Model/dq to 123 ==
  Idq : Inport
  w_ref : Inport  Port=2
  Add : Sum
  Clark KCInv : Constant  Value=inv(2/3*[1 -0.5 -0.5; 0 sqrt(3)/2 -sqrt(3)/2; 1/sqrt(2) 1/sqrt(2) 1/sqrt(2)])
  Constant : Constant  Value=[1 0; 0 1]
  Constant1 : Constant  Value=[0 -1; 1 0]
  Constant2 : Constant  Value=0
  Cos : Trigonometry  Operator=sincos
  Integrator : Integrator
  Mux : Mux  Inputs=2
  Product1 : Product
  Product2 : Product
  Product3 : Product  Multiplication=Matrix(*)
  Product5 : Product  Multiplication=Matrix(*)
  Selector : Selector  InputPortWidth=4  IndexOptions=Index vector (dialog)  Indices=[1 2]  OutputSizes=1
  Iab : Outport  VectorParamsAs1DForOutWhenUnconnected=off
  I123 : Outport  Port=2  VectorParamsAs1DForOutWhenUnconnected=off
  wires:
  Cos/1 -> Product1/2
  Constant1/1 -> Product1/1
  Product2/1 -> Add/2
  Cos/2 -> Product2/1
  Product1/1 -> Add/1
  Constant/1 -> Product2/2
  Add/1 -> Product3/1
  Idq/1 -> Selector/1
  Product3/1 -> Mux/1, Iab/1
  Clark KCInv/1 -> Product5/1
  Product5/1 -> I123/1
  Mux/1 -> Product5/2
  Constant2/1 -> Mux/2
  Selector/1 -> Product3/2
  Integrator/1 -> Cos/1
  w_ref/1 -> Integrator/1

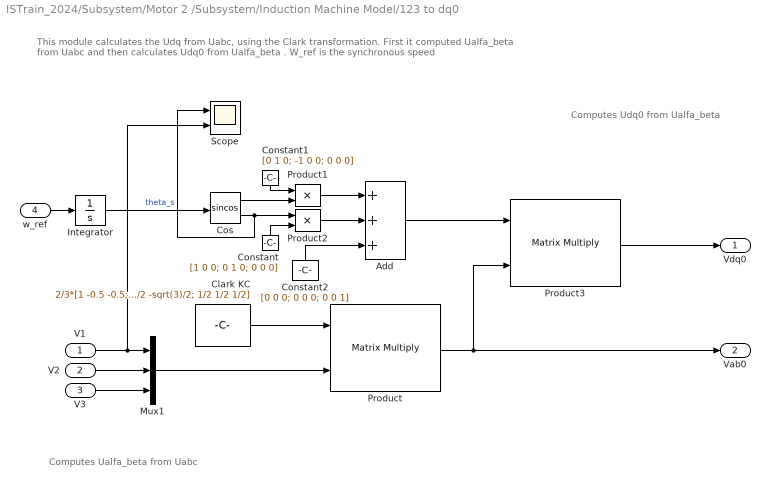
== system ISTrain_2024/Subsystem/Motor 2 /Subsystem/Induction Machine Model/123 to dq0 ==
  note: Computes Ualfa_beta from Uabc
  note: This module calculates the Udq from Uabc, using the Clark transformation.
      | First it computed Ualfa_beta from Uabc and then calculates Udq0 from Ualfa_beta .
      | W_ref is the synchronous speed
  note: Computes Udq0 from Ualfa_beta
  V1 : Inport
  V2 : Inport  Port=2
  V3 : Inport  Port=3
  w_ref : Inport  Port=4
  Add : Sum  Inputs=+++
  Clark KC : Constant  Value=2/3*[1 -0.5 -0.5; 0 sqrt(3)/2 -sqrt(3)/2; 1/2 1/2 1/2]
  Constant : Constant  Value=[1 0 0; 0 1 0; 0 0 0]
  Constant1 : Constant  Value=[0 1 0; -1 0 0; 0 0 0]
  Constant2 : Constant  Value=[0 0 0; 0 0 0; 0 0 1]
  Cos : Trigonometry  Operator=sincos
  Integrator : Integrator
  Mux1 : Mux  Inputs=3
  Product : Product  Multiplication=Matrix(*)
  Product1 : Product
  Product2 : Product
  Product3 : Product  Multiplication=Matrix(*)
  Scope : Scope  NumInputPorts=2
  Vdq0 : Outport  VectorParamsAs1DForOutWhenUnconnected=off
  Vab0 : Outport  Port=2  VectorParamsAs1DForOutWhenUnconnected=off
  wires:
  Clark KC/1 -> Product/1
  Mux1/1 -> Product/2
  Product/1 -> Product3/2, Vab0/1
  Integrator/1 -> Cos/1  "theta_s"
  Cos/1 -> Product1/2
  Constant1/1 -> Product1/1
  Cos/2 -> Scope/1, Product2/1
  Constant/1 -> Product2/2
  Product1/1 -> Add/1
  Product2/1 -> Add/2
  Add/1 -> Product3/1
  Product3/1 -> Vdq0/1
  w_ref/1 -> Integrator/1
  Constant2/1 -> Add/3
  V2/1 -> Mux1/2
  V3/1 -> Mux1/3
  V1/1 -> Mux1/1, Scope/2

== system ISTrain_2024/Subsystem/Motor 2 /Subsystem/Induction Machine Model/Eletromagnetic Torque ==
  Idq : Inport
  Constant : Constant  Value=3/2*LM*Pp
  Demux1 : Demux  Outputs=2
  Product : Product
  Product1 : Product  Inputs=1
  Product2 : Product  Inputs=1
  Selector : Selector  InputPortWidth=4  IndexOptions=Index vector (dialog)  Indices=[2 3 1 4]  OutputSizes=1
  Sum : Sum  Inputs=+-
  Te : Outport  VectorParamsAs1DForOutWhenUnconnected=off
  wires:
  Sum/1 -> Product/1
  Product1/1 -> Sum/1
  Demux1/1 -> Product1/1
  Product2/1 -> Sum/2
  Constant/1 -> Product/2
  Demux1/2 -> Product2/1
  Product/1 -> Te/1
  Idq/1 -> Selector/1
  Selector/1 -> Demux1/1

== system ISTrain_2024/Subsystem/Motor 2 /Subsystem/Induction Machine Model/State-Space Model ==
  Vdq : Inport
  W : Inport  Port=2
  Constant : Constant  Value=RLInv  VectorParams1D=off
  Constant1 : Constant  Value=[0;0]
  Integrator : Integrator
  Linv : Constant  Value=inv(LMatrix)  VectorParams1D=off
  Product : Product  Multiplication=Matrix(*)
  Product1 : Product  Multiplication=Matrix(*)
  Sum : Sum  Inputs=|--
  Sum1 : Sum  Inputs=|++
  Vector Concatenate : Concatenate
  Idq : Outport  VectorParamsAs1DForOutWhenUnconnected=off
  phidq : Outport  Port=2  VectorParamsAs1DForOutWhenUnconnected=off
  wires:
  W/1 -> Sum/1
  Product/1 -> Sum1/2
  Constant/1 -> Sum/2
  Integrator/1 -> phidq/1, Product1/2, Product/2
  Product1/1 -> Idq/1
  Sum1/1 -> Integrator/1
  Sum/1 -> Product/1
  Linv/1 -> Product1/1
  Vdq/1 -> Vector Concatenate/1
  Constant1/1 -> Vector Concatenate/2
  Vector Concatenate/1 -> Sum1/1

== system ISTrain_2024/Subsystem/Motor 2 /Subsystem/Induction Machine Model/W Matrix Computation ==
  note: computes W(dPsi/dt)=[0                     -d(theta_s)/dt          0                       0;
      |                                     d(theta_s)/dt           0                      0                      0;
      |                                    0                              0                      0             -d(theta_r)/dt;
      |                                    0                              0             d(theta_r)/dt              0;]
  w_ref : Inport
  wm : Inport  Port=2
  Gain : Gain  Gain=Pp
  Gain1 : Gain  Gain=-1  SaturateOnIntegerOverflow=on  OutDataTypeStr=Inherit: Same as input  ParamDataTypeStr=Inherit: Same as input
  Product : Product
  Sum2 : Sum  Inputs=-+|  InputSameDT=on  SaturateOnIntegerOverflow=on  OutDataTypeStr=Inherit: Same as first input
  W(3,4)=wr-1 : Assignment  NumberOfDimensions=2  IndexOptions=Index vector (dialog),Index vector (dialog)  Indices=3,4  OutputSizes=1,1
  W(4,3)=1-wr1 : Assignment  NumberOfDimensions=2  IndexOptions=Index vector (dialog),Index vector (dialog)  Indices=4,3  OutputSizes=1,1
  u1 : Constant  Value="[ 0 -1  0  0; 1  0  0  0;  0  0  0  0;  0  0  0  0]"
  W : Outport  InitialOutput=0  VectorParamsAs1DForOutWhenUnconnected=off
  wires:
  Gain1/1 -> W(3,4)=wr-1/2
  W(3,4)=wr-1/1 -> W/1
  Sum2/1 -> W(4,3)=1-wr1/2, Gain1/1  "we-w"
  wm/1 -> Gain/1
  W(4,3)=1-wr1/1 -> W(3,4)=wr-1/1
  Gain/1 -> Sum2/1
  w_ref/1 -> Product/1, Sum2/2
  u1/1 -> Product/2
  Product/1 -> W(4,3)=1-wr1/1

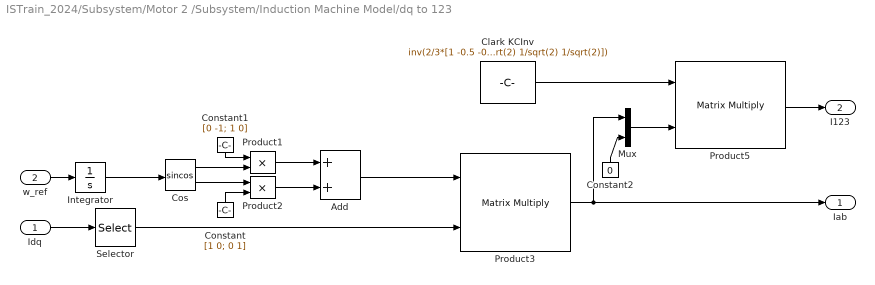
== system ISTrain_2024/Subsystem/Motor 2 /Subsystem/Induction Machine Model/dq to 123 ==
  Idq : Inport
  w_ref : Inport  Port=2
  Add : Sum
  Clark KCInv : Constant  Value=inv(2/3*[1 -0.5 -0.5; 0 sqrt(3)/2 -sqrt(3)/2; 1/sqrt(2) 1/sqrt(2) 1/sqrt(2)])
  Constant : Constant  Value=[1 0; 0 1]
  Constant1 : Constant  Value=[0 -1; 1 0]
  Constant2 : Constant  Value=0
  Cos : Trigonometry  Operator=sincos
  Integrator : Integrator
  Mux : Mux  Inputs=2
  Product1 : Product
  Product2 : Product
  Product3 : Product  Multiplication=Matrix(*)
  Product5 : Product  Multiplication=Matrix(*)
  Selector : Selector  InputPortWidth=4  IndexOptions=Index vector (dialog)  Indices=[1 2]  OutputSizes=1
  Iab : Outport  VectorParamsAs1DForOutWhenUnconnected=off
  I123 : Outport  Port=2  VectorParamsAs1DForOutWhenUnconnected=off
  wires:
  Cos/1 -> Product1/2
  Constant1/1 -> Product1/1
  Product2/1 -> Add/2
  Cos/2 -> Product2/1
  Product1/1 -> Add/1
  Constant/1 -> Product2/2
  Add/1 -> Product3/1
  Idq/1 -> Selector/1
  Product3/1 -> Mux/1, Iab/1
  Clark KCInv/1 -> Product5/1
  Product5/1 -> I123/1
  Mux/1 -> Product5/2
  Constant2/1 -> Mux/2
  Selector/1 -> Product3/2
  Integrator/1 -> Cos/1
  w_ref/1 -> Integrator/1

== matlab function ISTrain_2024/Subsystem/Alert_Zone/MATLAB Function ==
  data: SoC input; alert output; Voltage input; C_rate input
function alert = AlertZone(SoC, Voltage, C_rate)
% Throws an error if any alert condition is violated

% Thresholds
SoC_thresh = 0.10;
V_thresh   = 42;
C_thresh   = 3;

% Check conditions
if SoC < SoC_thresh
    error('ALERT: State of Charge dropped below 10%% (SoC = %.2f)', SoC);
elseif Voltage < V_thresh
    error('ALERT: Voltage dropped below minimum threshold (Voltage = %.2f V)', Voltage);
elseif C_rate > C_thresh
    error('ALERT: C-rate exceeded safe limit (C_rate = %.2f)', C_rate);
end

% No alert
alert = 0;
end

== matlab function ISTrain_2024/Subsystem/Primary Battery Systen/MATLAB Function ==
  data: P_in input; V_out output; I_out output; SoC_out output; C_out output; P_out output
function [V_out, I_out, SoC_out, C_out, P_out] = batteryModel(P_in)
% LiFePO4 Battery model (simplified steady-state)
% Assumes constant capacity and internal resistance

% === Parameters ===
persistent SoC_prev V_RC_prev

if isempty(SoC_prev)
    SoC_prev = 1.0;           % initial SoC (100%)
end
if isempty(V_RC_prev)
    V_RC_prev = 0;            % initial RC voltage
end

% Simulation settings
dt = 0.001;                       % 1-second step (adjust to match Simulink sample time)
R0 = 0.02;                    % internal resistance [Ohm]
R1 = 0.005;
C1 = 1000;                    % RC capacitance [F]
voc_min = 42;                 % cut-off voltage [V]

% Battery pack
cell_voltage = 24;            % V
num_series = 2;
num_parallel = 2;
cell_capacity = 100;           % Ah
V_oc_nom = cell_voltage * num_series;
pack_capacity_Ah = cell_capacity * num_parallel;        % 200 Ah
Q_total = pack_capacity_Ah * 3600; % Coulombs

% V_oc vs SoC approximation
SoC_points = linspace(0,1,11);
Voc_points = [24.0 25.2 25.4 25.6 25.7 25.8 25.9 26.0 26.2 26.4 26.8] * num_series;
V_oc = interp1(SoC_points, Voc_points, SoC_prev, 'linear', 'extrap');

% Limit power if voltage or SoC too low
if SoC_prev <= 0.1 || V_oc <= voc_min
    P_in = 0;
end

% Compute current
I = P_in / max(V_oc, 1e-3);

% RC voltage update
dV_RC = (-V_RC_prev + I * R1) / (R1 * C1) * dt;
V_RC_new = V_RC_prev + dV_RC;

% Terminal voltage
V_terminal = V_oc - I * R0 - V_RC_new;
if V_terminal < voc_min
    V_terminal = voc_min;
    I = 0;
    P_in = 0;
end

% Update SoC
dQ = I * dt;
Q_used = (1 - SoC_prev) * Q_total + dQ;
SoC_new = max(0, 1 - Q_used / Q_total);

% Outputs
V_out = V_terminal;
I_out = I;
SoC_out = SoC_new;
C_out = I / pack_capacity_Ah;  % C-rate
P_out = P_in;

% Update persistent vars
SoC_prev = SoC_new;
V_RC_prev = V_RC_new;
end

== matlab function ISTrain_2024/Subsystem/Dynamics/MATLAB Function ==
  data: m_total input; F_res output; g input; Crr input; grade input
function F_res = ComputeResistance(m_total, g, Crr, grade)
F_rr = m_total * g * Crr;
F_grade = m_total * g * grade;
F_res = F_rr + F_grade;
end
